simulink model "simulation_of_simple_pendulum_motion_without_damper"  (R2021a)
settings: Solver=VariableStepAuto  StartTime=0.0  StopTime=10.0  MaxStep=1e-3  RelTol=1e-3
settings Model: Creator=YasserNet  LastModifiedBy=YasserNet

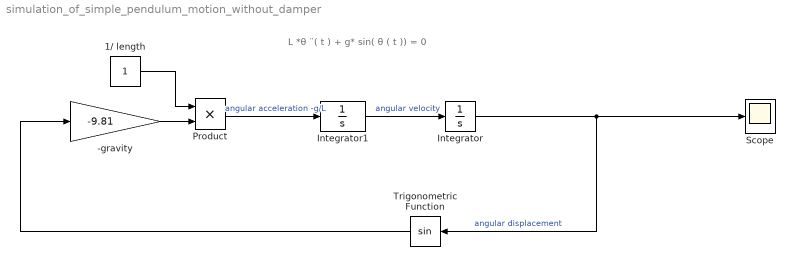
== system simulation_of_simple_pendulum_motion_without_damper ==
  note: L *θ ¨( t ) + g* sin( θ ( t )) = 0
  -gravity : Gain  Gain=-9.81  OutDataTypeStr=double
  1/ length : Constant
  Integrator : Integrator  InitialCondition=1
  Integrator1 : Integrator
  Product : Product
  Scope : Scope
  Trigonometric Function : Trigonometry
  wires:
  Integrator1/1 -> Integrator/1  "angular velocity"
  Integrator/1 -> Trigonometric Function/1, Scope/1  "angular displacement"
  -gravity/1 -> Product/2
  Trigonometric Function/1 -> -gravity/1
  1/ length/1 -> Product/1
  Product/1 -> Integrator1/1  "angular acceleration  -g/L"
